simulink model "W2Prob1"  (R2020b)
settings: Solver=VariableStepAuto  StartTime=0.0  StopTime=100  RelTol=1e-3
settings Model: EnablePacing=on  PacingRate=0.890000  Creator=deves  LastModifiedBy=deves

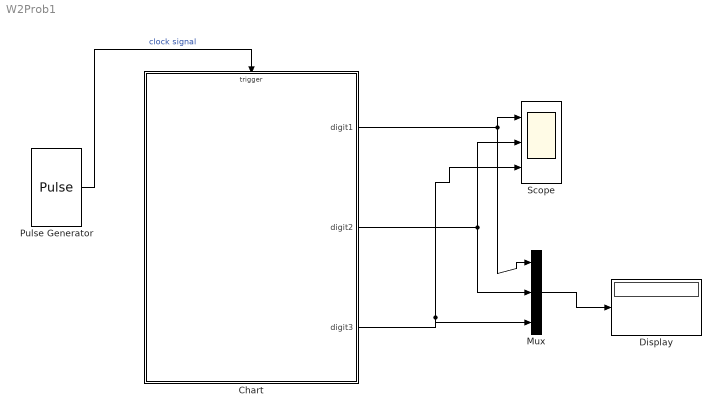
== system W2Prob1 ==
  Chart : Stateflow chart  TreatAsAtomicUnit=on
  Display : Display
  Mux : Mux  Inputs=3
  Pulse Generator : DiscretePulseGenerator  PulseType=Time based  Period=1  PulseWidth=5
  Scope : Scope  NumInputPorts=3
  wires:
  Chart/1(digit1) -> Mux/1, Scope/1
  Chart/2(digit2) -> Mux/2, Scope/2
  Chart/3(digit3) -> Scope/3, Mux/3
  Mux/1 -> Display/1
  Pulse Generator/1 -> Chart/Trigger  "clock signal"

== stateflow chart W2Prob1/Chart ==
  state Digit_2 [parallel]
    settings: executionOrder=2
    state count_0
      en:
      digit2=0;
    state count_1
      en:
      digit2=1;
    state count_2
      en:
      digit2=2;
    state count_3
      en:
      digit2=3;
    state count_4
      en:
      digit2=4;
    (default) -> Digit_2.count_0
    Digit_2.count_4 -> Digit_2.count_0 : d2{Digit_3.d3}
    Digit_2.count_0 -> Digit_2.count_1 : d2
    Digit_2.count_1 -> Digit_2.count_2 : d2
    Digit_2.count_2 -> Digit_2.count_3 : d2
    Digit_2.count_3 -> Digit_2.count_4 : d2
  state Digit_3 [parallel]
    settings: executionOrder=3
    state count_0
      en:
      digit3=0;
    state count_1
      en:
      digit3=1;
    state count_2
      en:
      digit3=2;
    state count_3
      en:
      digit3=3;
    state count_4
      en:
      digit3=4;
    (default) -> Digit_3.count_0
    Digit_3.count_4 -> Digit_3.count_0 : d3
    Digit_3.count_0 -> Digit_3.count_1 : d3
    Digit_3.count_1 -> Digit_3.count_2 : d3
    Digit_3.count_2 -> Digit_3.count_3 : d3
    Digit_3.count_3 -> Digit_3.count_4 : d3
  state Digit_1 [parallel]
    settings: executionOrder=1
    state count_0
      en:
      digit1=0;
    state count_1
      en:
      digit1=1;
    state count_2
      en:
      digit1=2;
    state count_3
      en:
      digit1=3;
    state count_4
      en:
      digit1=4;
    (default) -> Digit_1.count_0
    Digit_1.count_4 -> Digit_1.count_0 : clock{Digit_2.d2}
    Digit_1.count_0 -> Digit_1.count_1
    Digit_1.count_1 -> Digit_1.count_2 : clock
    Digit_1.count_2 -> Digit_1.count_3 : clock
    Digit_1.count_3 -> Digit_1.count_4 : clock
  data: digit1 output; digit2 output; digit3 output
  events: d2 local FUNCTION_CALL_EVENT; d3 local FUNCTION_CALL_EVENT; clock input RISING_EDGE_EVENT
